simulink model "ContactEstimationBlock"  (R2014a)
settings: Solver=ode45  StartTime=0.0  StopTime=10.0  RelTol=1e-3
undefined symbols (not defined in the file): fcut_contact, g, k_sea, m_total_real, sample_time
settings Model: Creator=wmartin  LastModifiedBy=wmartin

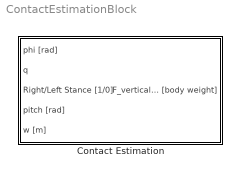
== system ContactEstimationBlock ==
  Contact Estimation : Subsystem

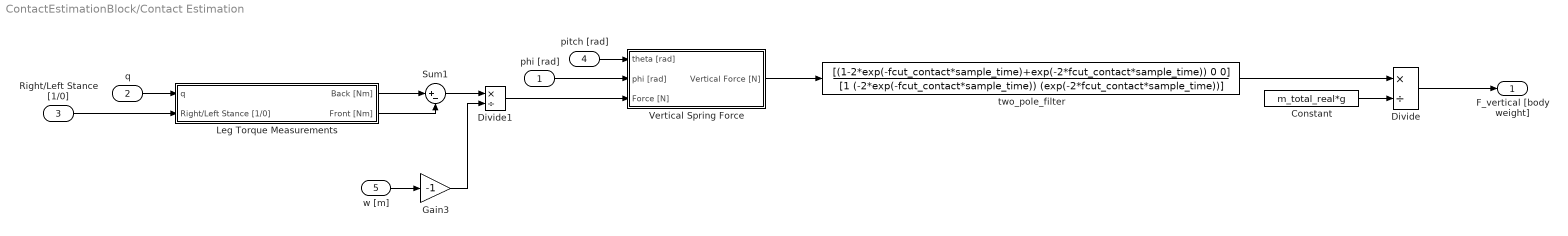
== system ContactEstimationBlock/Contact Estimation ==
  phi [rad] : Inport
  q : Inport  Port=2
  Right/Left Stance [1/0] : Inport  Port=3
  pitch [rad] : Inport  Port=4
  w [m] : Inport  Port=5
  Constant : Constant  Value=m_total_real*g
  Divide : Product  Inputs=*/
  Divide1 : Product  Inputs=*/
  Gain3 : Gain  Gain=-1
  Leg Torque Measurements : Subsystem
  Sum1 : Sum  Inputs=|+-
  Vertical Spring Force : Subsystem
  two_pole_filter : DiscreteTransferFcn  Numerator=[(1-2*exp(-fcut_contact*sample_time)+exp(-2*fcut_contact*sample_time)) 0 0]  Denominator=[1 (-2*exp(-fcut_contact*sample_time)) (exp(-2*fcut_contact*sample_time))]  SampleTime=sample_time
  F_vertical [body weight] : Outport
  wires:
  Vertical Spring Force/1(Vertical Force [N]) -> two_pole_filter/1
  Constant/1 -> Divide/2
  two_pole_filter/1 -> Divide/1
  q/1 -> Leg Torque Measurements/1(q)
  Leg Torque Measurements/1(Back [Nm]) -> Sum1/1
  Leg Torque Measurements/2(Front [Nm]) -> Sum1/2
  Sum1/1 -> Divide1/1
  Divide1/1 -> Vertical Spring Force/3(Force [N])
  pitch [rad]/1 -> Vertical Spring Force/1(theta [rad])
  w [m]/1 -> Gain3/1
  Gain3/1 -> Divide1/2
  phi [rad]/1 -> Vertical Spring Force/2(phi [rad])
  Divide/1 -> F_vertical [body weight]/1
  Right/Left Stance [1/0]/1 -> Leg Torque Measurements/2(Right/Left Stance [1/0])

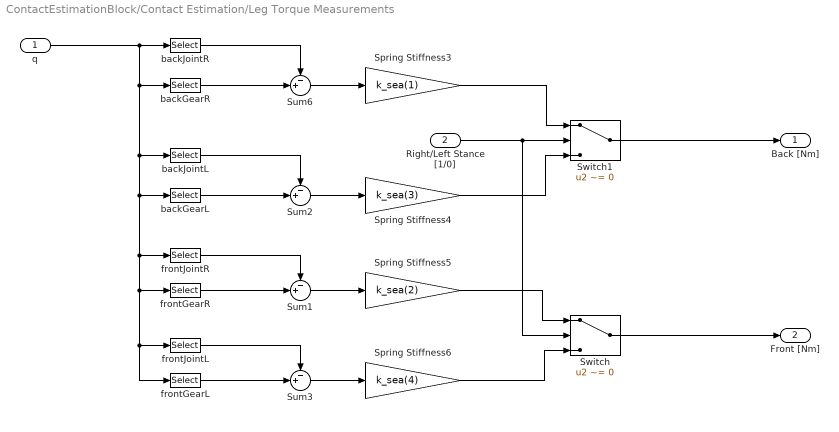
== system ContactEstimationBlock/Contact Estimation/Leg Torque Measurements ==
  q : Inport
  Right/Left Stance [1/0] : Inport  Port=2
  Spring Stiffness3 : Gain  Gain=k_sea(1)
  Spring Stiffness4 : Gain  Gain=k_sea(3)
  Spring Stiffness5 : Gain  Gain=k_sea(2)
  Spring Stiffness6 : Gain  Gain=k_sea(4)
  Sum{1..3,6} (4 alike) : Sum  Inputs=-+|
  Switch : Switch  Criteria=u2 ~= 0
  Switch1 : Switch  Criteria=u2 ~= 0
  backGearL : Selector  InputPortWidth=13  Indices=[6]
  backGearR : Selector  InputPortWidth=13  Indices=[2]
  backJointL : Selector  InputPortWidth=13  Indices=[5]
  backJointR : Selector  InputPortWidth=13  Indices=[1]
  frontGearL : Selector  InputPortWidth=13  Indices=[8]
  frontGearR : Selector  InputPortWidth=13  Indices=[4]
  frontJointL : Selector  InputPortWidth=13  Indices=[7]
  frontJointR : Selector  InputPortWidth=13  Indices=[3]
  Back [Nm] : Outport
  Front [Nm] : Outport  Port=2
  wires:
  Spring Stiffness6/1 -> Switch/3
  Spring Stiffness5/1 -> Switch/1
  Spring Stiffness4/1 -> Switch1/3
  Spring Stiffness3/1 -> Switch1/1
  q/1 -> backJointR/1, frontGearL/1, frontJointL/1, frontGearR/1, frontJointR/1, backGearL/1, backJointL/1, backGearR/1
  backGearR/1 -> Sum6/2
  frontJointR/1 -> Sum1/1
  frontGearR/1 -> Sum1/2
  backJointR/1 -> Sum6/1
  Switch/1 -> Front [Nm]/1
  Sum1/1 -> Spring Stiffness5/1
  Sum6/1 -> Spring Stiffness3/1
  backGearL/1 -> Sum2/2
  frontJointL/1 -> Sum3/1
  frontGearL/1 -> Sum3/2
  backJointL/1 -> Sum2/1
  Switch1/1 -> Back [Nm]/1
  Sum2/1 -> Spring Stiffness4/1
  Sum3/1 -> Spring Stiffness6/1
  Right/Left Stance [1/0]/1 -> Switch/2, Switch1/2

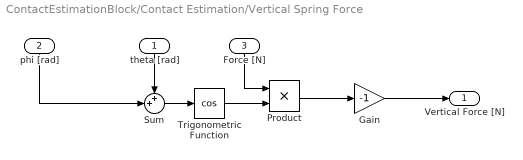
== system ContactEstimationBlock/Contact Estimation/Vertical Spring Force ==
  theta [rad] : Inport
  phi [rad] : Inport  Port=2
  Force [N] : Inport  Port=3
  Gain : Gain  Gain=-1
  Product : Product
  Sum : Sum  Inputs=++|
  Trigonometric Function : Trigonometry  Operator=cos
  Vertical Force [N] : Outport
  wires:
  Force [N]/1 -> Product/1
  phi [rad]/1 -> Sum/2
  theta [rad]/1 -> Sum/1
  Trigonometric Function/1 -> Product/2
  Product/1 -> Gain/1
  Sum/1 -> Trigonometric Function/1
  Gain/1 -> Vertical Force [N]/1
